simulink model "ex_1"  (R2018b)
settings: Solver=VariableStepAuto  StartTime=0.0  StopTime=10.0  RelTol=1e-3
values from neighbouring files (symbols this model uses):
  b = 8    [sitlab_2.m]
  f = 8    [sitlab_2.m]
  k = 16    [sitlab_2.m]
  m = 2    [sitlab_2.m]
settings Model: Creator=student  LastModifiedBy=Dell

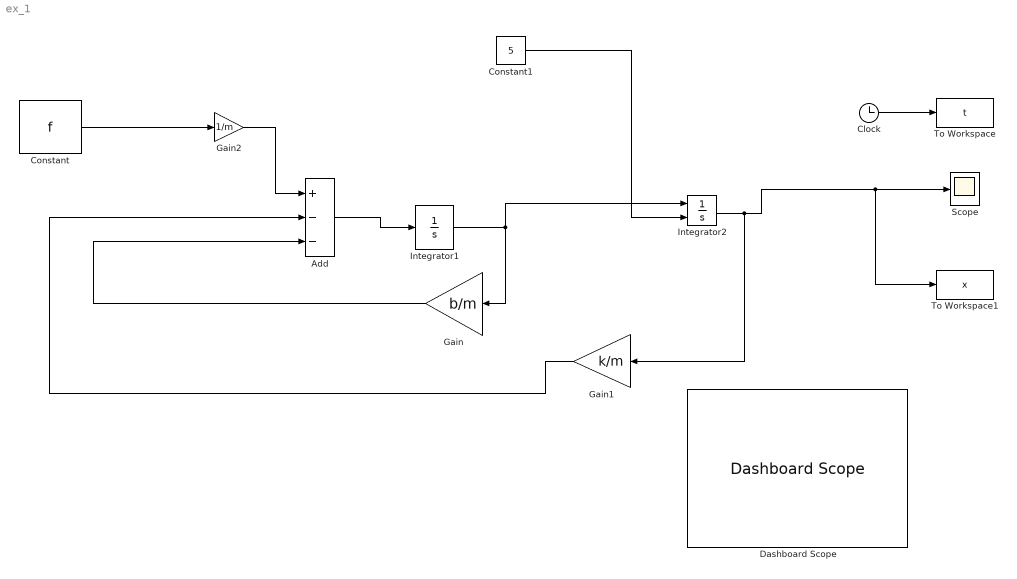
== system ex_1 ==
  Add : Sum  Inputs=+--
  Clock : Clock
  Constant : Constant  Value=f
  Constant1 : Constant  Value=5
  Dashboard Scope : DashboardScope  WebBlockId=9
  Gain : Gain  Gain=b/m
  Gain1 : Gain  Gain=k/m
  Gain2 : Gain  Gain=1/m
  Integrator1 : Integrator
  Integrator2 : Integrator  InitialConditionSource=external  InitialCondition=5
  Scope : Scope
  To Workspace : ToWorkspace  VariableName=t  SampleTime=-1
  To Workspace1 : ToWorkspace  VariableName=x  SampleTime=-1
  wires:
  Gain2/1 -> Add/1
  Gain1/1 -> Add/2
  Integrator2/1 -> To Workspace1/1, Scope/1, Gain1/1
  Constant/1 -> Gain2/1
  Gain/1 -> Add/3
  Add/1 -> Integrator1/1
  Integrator1/1 -> Integrator2/1, Gain/1
  Constant1/1 -> Integrator2/2
  Clock/1 -> To Workspace/1
